simulink model "notifbatreidroneM19"  (R2018a)
settings: Solver=VariableStepAuto  StartTime=0.0  StopTime=inf  RelTol=1e-3  EnableMultiTasking=on
settings Model: Creator=Ms  LastModifiedBy=syamsulfuad
settings OptimizationCC: LifeSpan=inf
settings DebuggingCC: SFUnexpectedBacktrackingDiag=warning  SFNoUnconditionalDefaultTransitionDiag=warning  SFExecutionAtInitializationDiag=none
settings CodeAppCC: StateflowObjectComments=on
settings GRTTargetCC: TargetLangStandard=C89/C90 (ANSI)  GeneratePreprocessorConditionals=Disable all
settings ConfigComp: CovMetricSettings=dw  CovHtmlReporting=on  CovSaveCumulativeToWorkspaceVar=on  CovSaveSingleToWorkspaceVar=on  CovExternalEMLEnable=off

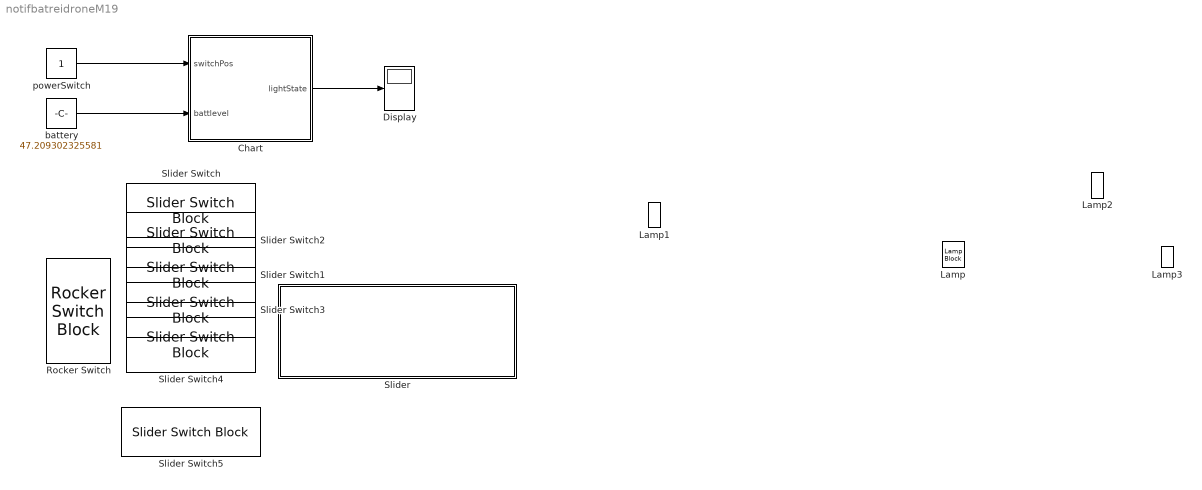
== system notifbatreidroneM19 ==
  Chart : Stateflow chart  TreatAsAtomicUnit=on
  Display : Display
  Lamp : LampBlock  WebBlockId=40  LabelPosition=Hide
  Lamp1 : LampBlock  WebBlockId=32  LabelPosition=Hide
  Lamp2 : LampBlock  WebBlockId=36  LabelPosition=Hide
  Lamp3 : LampBlock  WebBlockId=37  LabelPosition=Hide
  Rocker Switch : RockerSwitchBlock  WebBlockId=39
      settings: Values={{'Off', 'On'}, [0 1]}
  Slider : Subsystem  DialogController=hmiCreateDDGDialog  IsWebBlock=on  mask(MWDashboardBlock){webBlockId=6465138f-51e6-4dc9-adb4-8067bff19bad, webBlockType=slider, ShowInLibBrowser=on, ShowInitialText=on, HMISrcModelName=notifbatreidroneM18}
      mask prompts: webBlockId "WebBlock Id"; webBlockType "WebBlock Type"; HMISrcModelName "Source Model"
      mask Help: helpview([docroot '/mapfiles/simulink.map'], 'hmi_slider')
      mask Display:
      | if strcmp(get_param(bdroot(gcb),'BlockDiagramType'), 'library')
      |     image([(matlabroot) '/toolbox/simulink/hmi/icons/Slider.png']);
      | end
  Slider Switch : SliderSwitchBlock  WebBlockId=41  LabelPosition=Hide
      settings: Values={{'manual', 'auto pilot'}, [30 100]}
  Slider Switch1 : SliderSwitchBlock  WebBlockId=34  LabelPosition=Hide
      settings: Values={{'manual', 'A-MODE'}, [30 100]}
  Slider Switch2 : SliderSwitchBlock  WebBlockId=38  LabelPosition=Hide
      settings: Values={{'manual', 'P-MODE'}, [30 100]}
  Slider Switch3 : SliderSwitchBlock  WebBlockId=35  LabelPosition=Hide
      settings: Values={{'manual', 'F-MODE'}, [30 100]}
  Slider Switch4 : SliderSwitchBlock  WebBlockId=33  LabelPosition=Hide
      settings: Values={{'manual', 'S-MODE'}, [30 100]}
  Slider Switch5 : SliderSwitchBlock  WebBlockId=42  LabelPosition=Hide
      settings: Values={{'drop fps', 'high fps'}, [50 100]}
  battery : Constant  Value=47.209302325581
  powerSwitch : Constant
  wires:
  powerSwitch/1 -> Chart/1(switchPos)
  battery/1 -> Chart/2(battlevel)
  Chart/1(lightState) -> Display/1

== system notifbatreidroneM19/Slider ==

== stateflow chart notifbatreidroneM19/Chart ==
  state mode_manual
    state idle_check
      entry:
      refresh==1;
    state S_MODE
      entry:
      modeoff==1;
    state F_MODE
      entry:
      modeoff==1;
    state A_MODE
      entry:
      modeoff==1;
    state P_MODE
      entry:
      modeoff==1;
    state AutoPilot
      entry:
      modeauto==0;
    S_MODE -> (junction 91) : [manualmode==1]
    F_MODE -> (junction 91) : [manualmode==1]
    (junction 91) -> idle_check
    A_MODE -> (junction 91) : [manualmode==1]
    P_MODE -> (junction 91) : [manualmode==1]
    AutoPilot -> S_MODE [order 2] : [autooff==0]
    AutoPilot -> F_MODE [order 3] : [autooff==0]
    AutoPilot -> A_MODE [order 4] : [autooff==0]
    AutoPilot -> P_MODE [order 1] : [autooff==0]
  state mode_auto
    state AutoPilot1
      entry:
      modeauto=1;
    state S_MODE1
      entry:
      modeon==1;
    state F_MODE1
      entry:
      modeon==1;
    state A_MODE1
      entry:
      modeon==1;
    state P_MODE1
      entry:
      modeon==1;
    state Battery_high_performance
      entry:powerhigh==1;
    AutoPilot1 -> P_MODE1 [order 2] : [manualmode==0]
    AutoPilot1 -> A_MODE1 [order 3] : [manualmode==0]
    AutoPilot1 -> F_MODE1 [order 4] : [manualmode==0]
    AutoPilot1 -> S_MODE1 [order 1] : [manualmode==0]
    S_MODE1 -> Battery_high_performance : [autoon==1]
    F_MODE1 -> Battery_high_performance : [autoon==1]
    A_MODE1 -> Battery_high_performance : [autoon==1]
    P_MODE1 -> Battery_high_performance : [autoon==1]
  state OFF
    entry:
    lightState=0;
  state ON
    entry:
    lightState=1;
  state LiveCam
    entry:
    framefps<=60;
  state LOW_BATT
    entry:
    lightState=2;
  state LOW_BATT1
    entry:
    lightState=3;
  state LOW_BATT2
    entry:
    lightState=4;
  state EMPTY
    entry:
    lightState=4;
  (default) -> OFF [order 1]
  OFF -> ON : [switchPos==1]
  idle_check -> OFF : [lightState==0]
  ON -> (junction 22) [order 2] : [battlevel<=80]
  ON -> AutoPilot1 [order 3] : [switchup==1]
  (junction 22) -> LOW_BATT
  ON -> OFF [order 1] : [switchPos==0]
  LiveCam -> (junction 91) [order 1] : [fpsdrop==1]
  (junction 26) -> OFF
  EMPTY -> OFF : [switchPos==0]
  (junction 21) -> OFF : [battlevel>=50]
  (junction 11) -> OFF
  LiveCam -> EMPTY [order 2] : [battlevel<=10]
  LOW_BATT -> (junction 11) [order 1] : [battlevel>=80]
  LOW_BATT -> (junction 13) [order 2]
  Battery_high_performance -> (junction 13) : [battlevel>=50]
  (junction 97) -> LiveCam [order 1] : [criticallevel2<=1]
  (junction 97) -> LiveCam [order 2] : [criticallevel1<=1]
  (junction 13) -> LOW_BATT1 : [battlevel<=50]
  LOW_BATT1 -> (junction 21) [order 1]
  LOW_BATT1 -> (junction 27) [order 2]
  (junction 27) -> EMPTY [order 2] : [battlevel<=10]
  (junction 27) -> LOW_BATT2 [order 1] : [battlevel<=30]
  (default) -> (junction 97) [order 2] : [switchon==1]
  (junction 96) -> AutoPilot : [criticallevel2<=1]
  (default) -> (junction 96) [order 3] : [switchon==1]
  LOW_BATT2 -> (junction 26) : [battlevel>=30]
  data: switchPos input; battlevel input; lightState output; fps local int32; modeauto local; automodeon local; manualmodelon local
  events: autooff local FUNCTION_CALL_EVENT; fpsdrop local FUNCTION_CALL_EVENT; manualmode local FUNCTION_CALL_EVENT; switchup local FUNCTION_CALL_EVENT; modeoff local FUNCTION_CALL_EVENT; powerhigh local FUNCTION_CALL_EVENT; modeon local RISING_EDGE_EVENT; autoon local RISING_EDGE_EVENT; framefps local FUNCTION_CALL_EVENT; refresh local FUNCTION_CALL_EVENT; criticallevel local FUNCTION_CALL_EVENT; criticallevel1 local FUNCTION_CALL_EVENT; criticallevel2 local FUNCTION_CALL_EVENT; switchon local FUNCTION_CALL_EVENT
